simulink model "inc_enc_v26"  (R2023a)
settings: Solver=FixedStepDiscrete  StartTime=0.0  StopTime=SimulationsDauer  RelTol=1e-3
values from neighbouring files (symbols this model uses):
  CW_CCW_Switch = 0    [Init_IncreEncoder_v26.m]
  d_axis_hit_CompareValue = 125    [Init_IncreEncoder_v26.m]
  f_ISR = 40e3    (= 40000)    [Init_IncreEncoder_v26.m]
  IncPerTurn = 4100    [Init_IncreEncoder_v26.m]
  inital_zero_speed_timeout = speed_timeout_in_s*f_fpga    (= 5000)    [Init_IncreEncoder_v26.m]
  n_max = 6000    [Init_IncreEncoder_v26.m]
  Offset_Position_elec = 42    [Init_IncreEncoder_v26.m]
  Offset_Position_mech = 753    [Init_IncreEncoder_v26.m]
  OmegaPerOverSampl = 1500*((2*pi)/60)    (= 157.079632679)    [Init_IncreEncoder_v26.m]
  Periode = abs(1/Striche_pro_Sekunde)    [Init_IncreEncoder_v26.m]
  Phase_Delay_A = Periode/8    [Init_IncreEncoder_v26.m]
  Phase_Delay_B = -Periode/8    [Init_IncreEncoder_v26.m]
  PolePair = 10    [Init_IncreEncoder_v26.m]
  QuadratureFactor = 4    [Init_IncreEncoder_v26.m]
  reciprocal_iterations = 3    [Init_IncreEncoder_v26.m]
  T_fpga = 1/f_fpga    (= 1e-08)    [Init_IncreEncoder_v26.m]
  T_mech = 1e-08    [Init_IncreEncoder_v26.m]
undefined symbols (not defined in the file or in its folder): DiscIntNeverNeededParam
libraries: hdlsllib x4, dspsrcs4 x3, dspswit3 x2, spsEdgeDetectorLib x2, simulink_extras x1
(part 2 of 2)

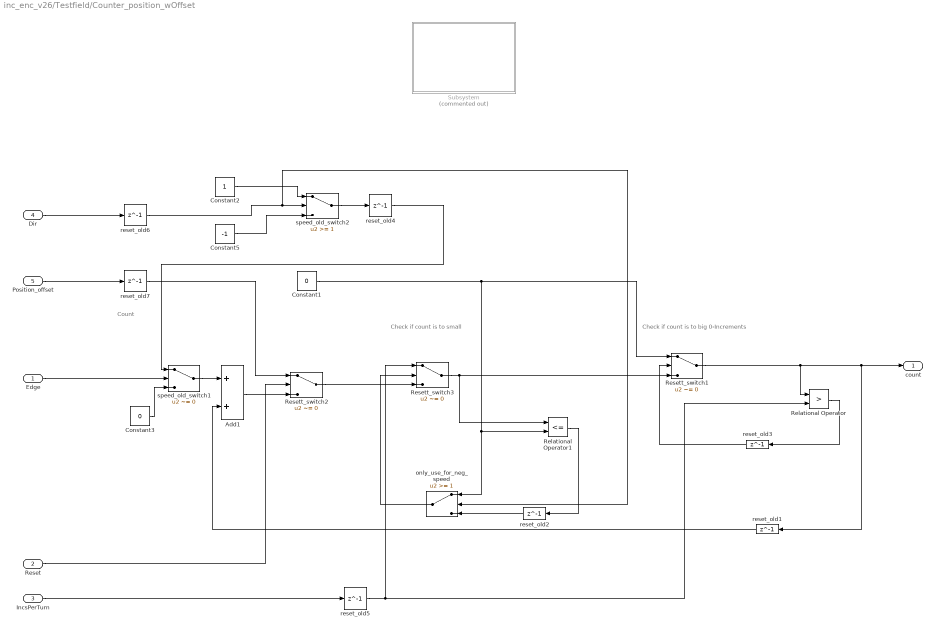
== system inc_enc_v26/Testfield/Counter_position_wOffset ==
  note: Check if count is to small
  note: Count
  note: Check if count is to big 0-Increments
  Edge : Inport
  Reset : Inport  Port=2
  IncsPerTurn : Inport  Port=3
  Dir : Inport  Port=4
  Position_offset : Inport  Port=5
  Add1 : Sum  AccumDataTypeStr=int16  OutDataTypeStr=int16
  Constant1 : Constant  Value=0  OutDataTypeStr=int16  SampleTime=-1
  Constant2 : Constant  OutDataTypeStr=int16  SampleTime=-1
  Constant3 : Constant  Value=0  OutDataTypeStr=int16  SampleTime=-1
  Constant5 : Constant  Value=-1  OutDataTypeStr=int16  SampleTime=-1
  Relational Operator : RelationalOperator  Operator=>  OutDataTypeStr=boolean  InputSameDT=off
  Relational Operator1 : RelationalOperator  Operator=<=  OutDataTypeStr=boolean  InputSameDT=off
  Resett_switch1 : Switch  Criteria=u2 ~= 0  OutDataTypeStr=uint16  SaturateOnIntegerOverflow=off  InputSameDT=off
  Resett_switch2 : Switch  Criteria=u2 ~= 0  OutDataTypeStr=int16  SaturateOnIntegerOverflow=off  InputSameDT=off
  Resett_switch3 : Switch  Criteria=u2 ~= 0  OutDataTypeStr=int16  SaturateOnIntegerOverflow=off  InputSameDT=off
  Subsystem : Subsystem  Commented=on
  only_use_for_neg_speed : Switch  Threshold=1  SaturateOnIntegerOverflow=off  InputSameDT=off
  reset_old{1..7} (7 alike) : Delay  DelayLength=1
  speed_old_switch1 : Switch  Criteria=u2 ~= 0  SaturateOnIntegerOverflow=off  InputSameDT=off
  speed_old_switch2 : Switch  Threshold=1  SaturateOnIntegerOverflow=off  InputSameDT=off
  count : Outport  VectorParamsAs1DForOutWhenUnconnected=off
  wires:
  speed_old_switch1/1 -> Add1/1
  Constant5/1 -> speed_old_switch2/3
  Relational Operator/1 -> reset_old3/1
  Constant2/1 -> speed_old_switch2/1
  reset_old4/1 -> speed_old_switch1/1
  reset_old5/1 -> Resett_switch3/1, Relational Operator/2
  Resett_switch2/1 -> Resett_switch3/3
  only_use_for_neg_speed/1 -> Resett_switch3/2
  Resett_switch3/1 -> Relational Operator1/1, Resett_switch1/3
  speed_old_switch2/1 -> reset_old4/1
  Relational Operator1/1 -> reset_old2/1
  reset_old3/1 -> Resett_switch1/2
  Resett_switch1/1 -> Relational Operator/1, count/1, reset_old1/1
  Constant1/1 -> only_use_for_neg_speed/1, Relational Operator1/2, Resett_switch1/1
  Constant3/1 -> speed_old_switch1/3
  IncsPerTurn/1 -> reset_old5/1
  Reset/1 -> Resett_switch2/2
  reset_old2/1 -> only_use_for_neg_speed/3
  Edge/1 -> speed_old_switch1/2
  reset_old1/1 -> Add1/2
  Position_offset/1 -> reset_old7/1
  Add1/1 -> Resett_switch2/3
  Dir/1 -> reset_old6/1
  reset_old6/1 -> only_use_for_neg_speed/2, speed_old_switch2/2
  reset_old7/1 -> Resett_switch2/1

== system inc_enc_v26/Testfield/Index_Latch ==
  Reset_in : Inport
  Constant : Constant  OutDataTypeStr=boolean
  Constant4 : Constant  Value=0  OutDataTypeStr=boolean
  Delay : Delay  DelayLength=1
  OR : Logic  Operator=OR  AllPortsSameDT=off  OutDataTypeStr=boolean
  Switch : Switch  Criteria=u2 > Threshold  SaturateOnIntegerOverflow=off  InputSameDT=off
  Index_found : Outport
  wires:
  Constant4/1 -> Switch/3
  Delay/1 -> OR/2
  Constant/1 -> Switch/1
  Switch/1 -> Index_found/1, Delay/1
  Reset_in/1 -> OR/1
  OR/1 -> Switch/2

== system inc_enc_v26/Create_Referenz/IncrementalEncoder_Floating/CutTheta_0_2PI ==
  In1 : Inport
  Add7 : Sum  Inputs=+-  OutDataTypeStr=double
  Gain : Gain  Gain=1/(2*pi)
  Gain11 : Gain  Gain=2*pi
  Rounding Function : Rounding
  Out1 : Outport  VectorParamsAs1DForOutWhenUnconnected=off
  wires:
  Gain/1 -> Rounding Function/1
  Rounding Function/1 -> Gain11/1
  Gain11/1 -> Add7/2
  In1/1 -> Gain/1, Add7/1
  Add7/1 -> Out1/1

== system inc_enc_v26/Create_Referenz/IncrementalEncoder_Floating/n_aus_theta_v4 ==
  theta : Inport
  Abs : Abs  SaturateOnIntegerOverflow=off
  Add : Sum  Inputs=-+
  Add1 : Sum  Inputs=+-
  Gain : Gain  Gain=2*pi
  Gain1 : Gain  Gain=1/T_mech
  Gain2 : Gain  Gain=60/(2*pi)
  Geschwindigkeitsfilter1 : Subsystem
  Rate Limiter2 1/T : RateLimiter  RisingSlewLimit=1/T_mech*10  FallingSlewLimit=-1/T_mech*10  SampleTimeMode=inherited
  Saturation : Saturate  UpperLimit=n_max  LowerLimit=-n_max
  Scope1 : Scope  NumInputPorts=5
  Scope2 : Scope  NumInputPorts=5
  Sign : Signum
  Switch : Switch  Threshold=3  SaturateOnIntegerOverflow=off  InputSameDT=off
  Unit Delay : UnitDelay  SampleTime=-1  HasFrameUpgradeWarning=on
  n : Outport  VectorParamsAs1DForOutWhenUnconnected=off
  wires:
  Switch/1 -> Scope1/3, Gain1/1
  Add/1 -> Scope2/1, Switch/1
  Gain/1 -> Add/1
  Sign/1 -> Gain/1
  Add1/1 -> Scope2/3, Add/2, Abs/1, Scope2/2, Switch/3, Sign/1
  Abs/1 -> Scope1/4, Switch/2
  Gain1/1 -> Scope1/2, Gain2/1
  theta/1 -> Scope2/5, Add1/1, Unit Delay/1
  Unit Delay/1 -> Scope2/4, Add1/2
  Gain2/1 -> Saturation/1
  Geschwindigkeitsfilter1/1(Out1) -> Scope1/5, Rate Limiter2 1/T/1
  Rate Limiter2 1/T/1 -> n/1
  Saturation/1 -> Scope1/1, Geschwindigkeitsfilter1/1(In1)

== system inc_enc_v26/IncEnc_V26/Counter_Theta_el_wOffset/Subsystem ==
  Add1 : Sum  AccumDataTypeStr=int16  OutDataTypeStr=int16
  Constant3 : Constant  Value=0  OutDataTypeStr=int16  SampleTime=-1
  Generate_Increment : Subsystem
  Resett_switch2 : Switch  Criteria=u2 ~= 0  OutDataTypeStr=int16  SaturateOnIntegerOverflow=off  InputSameDT=off
  reset_old6 : Delay  DelayLength=1
  speed_old_switch1 : Switch  Criteria=u2 ~= 0  SaturateOnIntegerOverflow=off  InputSameDT=off
  wires:
  ? -> speed_old_switch1/2
  ? -> Resett_switch2/2
  ? -> reset_old6/1
  ? -> Add1/2
  Generate_Increment/1(Increment) -> speed_old_switch1/1
  Resett_switch2/1 -> ?
  Constant3/1 -> speed_old_switch1/3
  ? -> Generate_Increment/1(Dir_in)
  reset_old6/1 -> Resett_switch2/1
  Add1/1 -> Resett_switch2/3
  speed_old_switch1/1 -> Add1/1

== system inc_enc_v26/IncEnc_V26/Counter_position_wOffset/Subsystem ==
  Add1 : Sum  AccumDataTypeStr=int16  OutDataTypeStr=int16
  Constant3 : Constant  Value=0  OutDataTypeStr=int16  SampleTime=-1
  Generate_Increment : Subsystem
  Resett_switch2 : Switch  Criteria=u2 ~= 0  OutDataTypeStr=int16  SaturateOnIntegerOverflow=off  InputSameDT=off
  reset_old6 : Delay  DelayLength=1
  speed_old_switch1 : Switch  Criteria=u2 ~= 0  SaturateOnIntegerOverflow=off  InputSameDT=off
  wires:
  speed_old_switch1/1 -> Add1/1
  Add1/1 -> Resett_switch2/3
  reset_old6/1 -> Resett_switch2/1
  ? -> Generate_Increment/1(Dir_in)
  Constant3/1 -> speed_old_switch1/3
  Resett_switch2/1 -> ?
  Generate_Increment/1(Increment) -> speed_old_switch1/1
  ? -> Add1/2
  ? -> reset_old6/1
  ? -> Resett_switch2/2
  ? -> speed_old_switch1/2

== system inc_enc_v26/IncEnc_V26/speed1/Average ==
  note: average 4 parallel measurements
  note: moving average of 4 last measurements, which in total results in a moving average of the last 8 samples
  "OmegaIn " : Inport
  NewMeasurement : Inport  Port=2
  DelayToCompensate_sum : Delay  DelayLength=1
  Demux2 : Demux
  Gain : Gain  Gain=1/4  OutDataTypeStr=fixdt(1,24,11)
  Gain1 : Gain  Gain=1/4  OutDataTypeStr=fixdt(1,24,11)
  Sum of Elements{1..6} (6 alike) : Sum  Inputs=2
  Unit Delay Enabled Synchronous : hdlsllib/Discrete/Unit Delay Enabled Synchronous  InitialCondition=0  SampleTime=-1
  Unit Delay Enabled Synchronous1 : hdlsllib/Discrete/Unit Delay Enabled Synchronous  InitialCondition=0  SampleTime=-1
  Unit Delay Enabled Synchronous2 : hdlsllib/Discrete/Unit Delay Enabled Synchronous  InitialCondition=0  SampleTime=-1
  delay : Delay  DelayLength=1
  delay1 : Delay  DelayLength=1
  Omega : Outport  VectorParamsAs1DForOutWhenUnconnected=off
  OmegaOut_MA_N4 : Outport  Port=2  VectorParamsAs1DForOutWhenUnconnected=off
  wires:
  Gain/1 -> OmegaOut_MA_N4/1  "omega moving average"
  DelayToCompensate_sum/1 -> Unit Delay Enabled Synchronous/1, delay1/1, Omega/1  "x(k)"
  Unit Delay Enabled Synchronous/1 -> Sum of Elements1/2, Unit Delay Enabled Synchronous1/1  "omega_delay1"
  Sum of Elements1/1 -> Sum of Elements3/1
  Sum of Elements3/1 -> Gain/1
  Unit Delay Enabled Synchronous2/1 -> Sum of Elements2/2  "omega_delay3"
  delay1/1 -> Sum of Elements1/1  "x(k)_1delayed"
  NewMeasurement/1 -> delay/1
  Sum of Elements2/1 -> Sum of Elements3/2
  delay/1 -> Unit Delay Enabled Synchronous/2, Unit Delay Enabled Synchronous1/2, Unit Delay Enabled Synchronous2/2  "enable_delayed"
  Unit Delay Enabled Synchronous1/1 -> Unit Delay Enabled Synchronous2/1, Sum of Elements2/1  "omega_delay2"
  Demux2/4 -> Sum of Elements5/2
  Demux2/3 -> Sum of Elements5/1
  Demux2/1 -> Sum of Elements4/1
  Sum of Elements5/1 -> Sum of Elements6/2
  Sum of Elements4/1 -> Sum of Elements6/1
  Demux2/2 -> Sum of Elements4/2
  Gain1/1 -> DelayToCompensate_sum/1  "omega summed 1/4"
  Sum of Elements6/1 -> Gain1/1
  "OmegaIn "/1 -> Demux2/1  "x(k)"

== system inc_enc_v26/IncEnc_V26/speed1/OS_factor_logic ==
  new_transisiton : Inport  PortDimensions=4
  Allow_ToCheckOversampling : Inport  Port=2
  state_edges : Inport  Port=3
  omega : Inport  Port=4
  OverSamplOmega : Inport  Port=5
  Abs : Abs  SaturateOnIntegerOverflow=off
  Constant : Constant  Commented=on  Value=[0,0,0,0]  OutDataTypeStr=boolean  SampleTime=T_fpga
  Data Type Conversion1 : DataTypeConversion  OutDataTypeStr=uint16  SaturateOnIntegerOverflow=off  RndMeth=Floor
  Delay1 : Delay  DelayLength=1  InitialCondition=0
  Delay6 : Delay  DelayLength=1  InitialCondition=0
  Delay7 : Delay  DelayLength=1  InitialCondition=1
  Sum : Sum  Inputs=+|-  AccumDataTypeStr=uint16
  align_oversamples : MATLAB Function  TreatAsAtomicUnit=on
  oversample_factor : MATLAB Function  TreatAsAtomicUnit=on
  oversampling_adjusted : Outport  PortDimensions=4
  oversampling_state : Outport  Port=2
  wires:
  OverSamplOmega/1 -> oversample_factor/3(OverSamplOmega)
  oversample_factor/1(state_Out) -> Delay7/1  "oversampling state Out"
  omega/1 -> Abs/1
  oversample_factor/2(InternalOmega_Out) -> Delay6/1
  Delay6/1 -> oversample_factor/5(InternalOmega)
  Abs/1 -> oversample_factor/2(ReadBack_Omega)
  Allow_ToCheckOversampling/1 -> oversample_factor/1(AllowCheckOverSampl)  "Allow_ToCheckOversampling"
  Delay7/1 -> Sum/1, align_oversamples/1(oversampling_factor), oversample_factor/4(state), Data Type Conversion1/1
  Data Type Conversion1/1 -> oversampling_state/1
  align_oversamples/1(delay_output) -> Delay1/1  "delay_output"
  new_transisiton/1 -> align_oversamples/2(new_transition)  "new_transistions"
  state_edges/1 -> align_oversamples/3(states)  "states"
  Sum/1 -> oversampling_adjusted/1
  Delay1/1 -> Sum/2

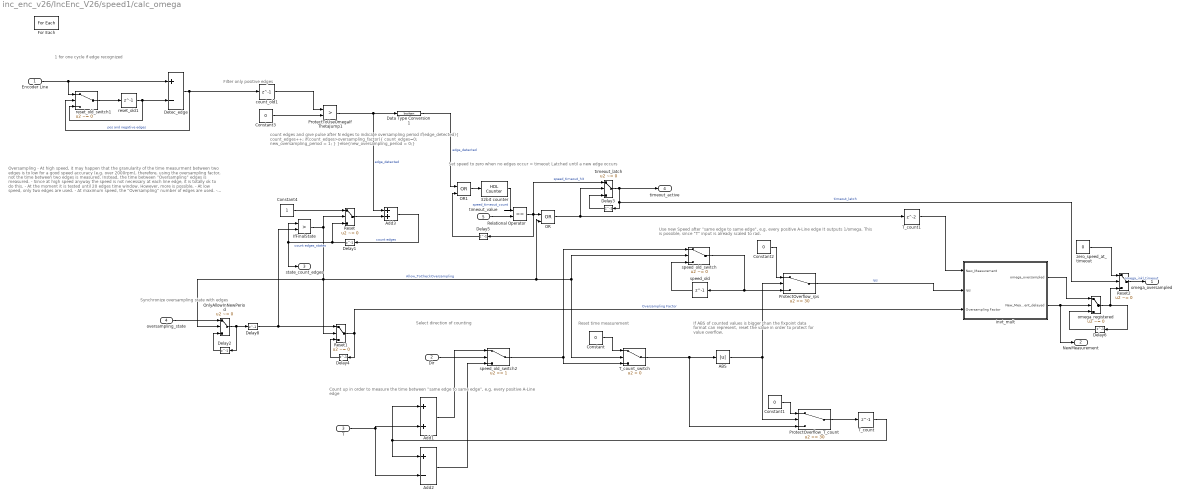
== system inc_enc_v26/IncEnc_V26/speed1/calc_omega ==
  note: Oversampling
      | - At high speed, it may happen that the granularity of the time measurment between
      | two edges is to low for a good speed accuracy (e.g. over 2000rpm), therefore, using
      | the oversampling factor, not the time between two edges is measured. Instead, the
      | time between "Oversampling" edges is measured.
      | - Since at high speed anyway the speed is not necessary at each line edge,
      |  it is totally ok to do this.
      | - At the moment it is tested until 20 edges time window. However, more is possible.
      | - At low speed, only two edges are used.
      | - At maximum speed, the "Oversampling" number of edges are used.
      | - Between them, a linear factor is used.
      | - Using the OverSampling number also at low speed is not possible,
      |  since the fixpoint range must be quite high! (fixdt(1,36,30) is used at the moment)
  note: Count up in order to measure the time between "same edge to same edge", e.g. every positive A-Line edge
  note: Reset time measurement
  note: 1 for one cycle if edge recognized
  note: Use new Speed after "same edge to same edge", e.g. every positive A-Line edge
      | It outputs 1/omega. This is possible, since "T" input is already scaled to rad.
  note: Select direction of counting
  note: If ABS of counted values is bigger than the
      | fixpoint data format can represent, reset the
      | value in order to protect for value overflow.
  note: Filter only positive edges
  note: count edges and give pulse after N edges to indicate oversampling period
      | if(edge_detected){
      | 	count_edges++;
      | 	if(count_edges>oversampling_factor){
      | 		count_edges=0;
      | 		new_oversampling_period = 1;
      | 	}
      | }else{new_oversampling_period = 0;}
  note: Synchronize oversampling state with edges
  note: Set speed to zero when no edges occur = timeout
      | Latched until a new edge occurs
  Encoder Line : Inport  Partition=on  PartitionDimension=1  PartitionWidth=1  PartitionOffset=0
  Dir : Inport  Port=2
  T : Inport  Port=3
  oversampling_state : Inport  Port=4  Partition=on  PartitionDimension=1  PartitionWidth=1  PartitionOffset=0
  timeout_value : Inport  Port=5  OutDataTypeStr=uint32
  32bit counter : hdlsllib/Sources/HDL Counter  CountType=Free running  CountInit=0  CountStep=1  CountMax=inital_zero_speed_timeout  CountFromType=Initial value  CountFrom=0  CountResetPort=on  CountLoadPort=off  CountEnbPort=off  CountDirPort=off  CountHitOutputPort=off  CountDataType=Unsigned  CountWordLen=32  CountFracLen=0  CountSampTime=1
  ABS : Abs  SaturateOnIntegerOverflow=off
  Add1 : Sum  OutDataTypeStr=Inherit: Same as first input
  Add2 : Sum  Inputs=+-  OutDataTypeStr=Inherit: Same as first input
  Add3 : Sum  OutDataTypeStr=Inherit: Same as accumulator
  Constant : Constant  Value=0  OutDataTypeStr=fixdt(1,38,32)  SampleTime=-1
  Constant1 : Constant  Value=0  OutDataTypeStr=fixdt(1,38,32)  SampleTime=-1
  Constant2 : Constant  Value=0  OutDataTypeStr=fixdt(1,38,32)  SampleTime=-1
  Constant3 : Constant  Value=0  OutDataTypeStr=int8  SampleTime=-1
  Constant4 : Constant  OutDataTypeStr=int8  SampleTime=-1
  Data Type Conversion1 : DataTypeConversion  OutDataTypeStr=boolean  SaturateOnIntegerOverflow=off  RndMeth=Floor
  Delay{1..6,8} (7 alike) : Delay  DelayLength=1  InitialCondition=0
  Detec_edge : Sum  Inputs=+-  AccumDataTypeStr=int8  OutDataTypeStr=int8
  For Each : ForEach  DisableCoverage=on
  IfFinalState : RelationalOperator  Operator=>  OutDataTypeStr=boolean  InputSameDT=off
  OR : Logic  Operator=OR  IconShape=distinctive  AllPortsSameDT=off  OutDataTypeStr=boolean
  OR1 : Logic  Operator=OR  IconShape=distinctive  AllPortsSameDT=off  OutDataTypeStr=boolean
  OnlyAllowInNewPeriod : Switch  Criteria=u2 ~= 0  Threshold=0.5  OutDataTypeStr=fixdt(0,16,0)  SaturateOnIntegerOverflow=off  InputSameDT=off
  ProtectOverflow_T_count : Switch  Threshold=30  SaturateOnIntegerOverflow=off  InputSameDT=off
  ProtectOverflow_rps : Switch  Threshold=30  OutDataTypeStr=fixdt(1,38,32)  SaturateOnIntegerOverflow=off  InputSameDT=off
  ProtectToUseOmegaIfThetaJump1 : RelationalOperator  Operator=>  OutDataTypeStr=fixdt(1,16)  InputSameDT=off
  Relational Operator : RelationalOperator  Operator===  OutDataTypeStr=boolean  RndMeth=Simplest  InputSameDT=off
  Reset : Switch  Criteria=u2 ~= 0  Threshold=0.5  OutDataTypeStr=fixdt(1,24,11)  SaturateOnIntegerOverflow=off  InputSameDT=off
  Reset1 : Switch  Criteria=u2 ~= 0  Threshold=0.5  OutDataTypeStr=Inherit: Inherit via back propagation  SaturateOnIntegerOverflow=off  InputSameDT=off
  Reset2 : Switch  Criteria=u2 ~= 0  Threshold=0.5  OutDataTypeStr=Inherit: Inherit via back propagation  SaturateOnIntegerOverflow=off  InputSameDT=off
  T_count : Delay  DelayLength=1
  T_count1 : Delay
  T_count_switch : Switch  Criteria=u2 > Threshold  SaturateOnIntegerOverflow=off  InputSameDT=off
  count_old1 : Delay  DelayLength=1
  invt_mult : Subsystem
  omega_registered : Switch  Criteria=u2 ~= 0  Threshold=0.5  SaturateOnIntegerOverflow=off  InputSameDT=off
  reset_old1 : Delay  DelayLength=1
  reset_old_switch1 : Switch  Criteria=u2 ~= 0  SaturateOnIntegerOverflow=off  InputSameDT=off
  speed_old : Delay  DelayLength=1
  speed_old_switch : Switch  Criteria=u2 ~= 0  OutDataTypeStr=fixdt(1,38,32)  SaturateOnIntegerOverflow=off  InputSameDT=off
  speed_old_switch2 : Switch  Threshold=1  SaturateOnIntegerOverflow=off  InputSameDT=off
  timeout_latch : Switch  Criteria=u2 ~= 0  Threshold=0.5  OutDataTypeStr=Inherit: Inherit via back propagation  SaturateOnIntegerOverflow=off  InputSameDT=off
  zero_speed_at_timeout : Constant  Value=0  OutDataTypeStr=fixdt(1,24,11)  SampleTime=-1
  omega_oversampled : Outport  ConcatenationDimension=1  VectorParamsAs1DForOutWhenUnconnected=off
  NewMeasurement : Outport  Port=2  ConcatenationDimension=1  VectorParamsAs1DForOutWhenUnconnected=off
  state_count_edges : Outport  Port=3  ConcatenationDimension=1  VectorParamsAs1DForOutWhenUnconnected=off
  timeout_active : Outport  Port=4  OutDataTypeStr=boolean  ConcatenationDimension=1  VectorParamsAs1DForOutWhenUnconnected=off
  wires:
  Constant/1 -> T_count_switch/1
  Constant1/1 -> ProtectOverflow_T_count/1
  Constant2/1 -> ProtectOverflow_rps/1
  speed_old_switch/1 -> ProtectOverflow_rps/3, speed_old/1
  speed_old/1 -> speed_old_switch/3
  T/1 -> Add1/2, Add2/2
  ProtectOverflow_T_count/1 -> T_count/1
  T_count/1 -> Add2/1, Add1/1
  speed_old_switch2/1 -> speed_old_switch/1, T_count_switch/3
  count_old1/1 -> ProtectToUseOmegaIfThetaJump1/1
  Constant3/1 -> ProtectToUseOmegaIfThetaJump1/2
  Encoder Line/1 -> reset_old_switch1/1, Detec_edge/1
  reset_old_switch1/1 -> reset_old1/1
  reset_old1/1 -> reset_old_switch1/3, Detec_edge/2
  Detec_edge/1 -> reset_old_switch1/2, count_old1/1  "pos and negative edges"
  Dir/1 -> speed_old_switch2/2
  Add1/1 -> speed_old_switch2/1
  Add2/1 -> speed_old_switch2/3
  T_count_switch/1 -> ABS/1, ProtectOverflow_T_count/3
  ABS/1 -> ProtectOverflow_T_count/2, ProtectOverflow_rps/2
  IfFinalState/1 -> OR/2, speed_old_switch/2, T_count_switch/2, Reset1/2, OnlyAllowInNewPeriod/2, Reset/2  "Allow_ToCheckOversampling"
  OnlyAllowInNewPeriod/1 -> Delay2/1, Delay8/1
  Delay1/1 -> Reset/3, state_count_edges/1, IfFinalState/1  "count edges_states"
  Add3/1 -> Delay1/1  "count edges"
  Reset/1 -> Add3/2
  Constant4/1 -> Reset/1
  Reset1/1 -> invt_mult/3(Oversampling Factor), Delay4/1  "Oversampling Factor"
  Delay2/1 -> OnlyAllowInNewPeriod/3
  oversampling_state/1 -> OnlyAllowInNewPeriod/1
  Delay4/1 -> Reset1/3
  Delay8/1 -> Reset1/1, IfFinalState/2
  ProtectToUseOmegaIfThetaJump1/1 -> Add3/1, Data Type Conversion1/1  "edge_detected"
  Relational Operator/1 -> Delay5/1, OR/1, timeout_latch/1  "speed_timeout_hit"
  zero_speed_at_timeout/1 -> Reset2/1
  Reset2/1 -> omega_oversampled/1  "omega_inkl_timeout"
  timeout_latch/1 -> timeout_active/1, Delay3/1, Reset2/2  "timeout_latch"
  Delay3/1 -> timeout_latch/3
  Data Type Conversion1/1 -> OR1/1  "edge_detected"
  timeout_value/1 -> Relational Operator/2
  32bit counter/1 -> Relational Operator/1  "speed_timeout_count"
  OR1/1 -> 32bit counter/1
  Delay5/1 -> OR1/2
  omega_registered/1 -> Reset2/3, Delay6/1
  Delay6/1 -> omega_registered/3
  OR/1 -> T_count1/1, timeout_latch/2
  ProtectOverflow_rps/1 -> invt_mult/2(rps)  "rps"
  invt_mult/1(omega_oversampled) -> omega_registered/1
  invt_mult/2(New_Measurement_delayed) -> NewMeasurement/1, omega_registered/2
  T_count1/1 -> invt_mult/1(New_Measurement)

== system inc_enc_v26/Testfield/Counter_position_wOffset/Subsystem ==
  Add1 : Sum  AccumDataTypeStr=int16  OutDataTypeStr=int16
  Constant3 : Constant  Value=0  OutDataTypeStr=int16  SampleTime=-1
  Generate_Increment : Subsystem
  Resett_switch2 : Switch  Criteria=u2 ~= 0  OutDataTypeStr=int16  SaturateOnIntegerOverflow=off  InputSameDT=off
  reset_old6 : Delay  DelayLength=1
  speed_old_switch1 : Switch  Criteria=u2 ~= 0  SaturateOnIntegerOverflow=off  InputSameDT=off
  wires:
  speed_old_switch1/1 -> Add1/1
  Add1/1 -> Resett_switch2/3
  reset_old6/1 -> Resett_switch2/1
  ? -> Generate_Increment/1(Dir_in)
  Constant3/1 -> speed_old_switch1/3
  Resett_switch2/1 -> ?
  Generate_Increment/1(Increment) -> speed_old_switch1/1
  ? -> Add1/2
  ? -> reset_old6/1
  ? -> Resett_switch2/2
  ? -> speed_old_switch1/2

== system inc_enc_v26/Create_Referenz/IncrementalEncoder_Floating/n_aus_theta_v4/Geschwindigkeitsfilter1 ==
  In1 : Inport
  Add1 : Sum  Inputs=+-
  Discrete-Time Integrator2 : DiscreteIntegrator  SampleTime=-1  ICPrevOutput=DiscIntNeverNeededParam  ICPrevScaledInput=DiscIntNeverNeededParam
  Gain2 2500 10000 : Gain  Gain=10000
  Scope1 : Scope  NumInputPorts=5
  Out1 : Outport  InitialOutput=[0]  VectorParamsAs1DForOutWhenUnconnected=off
  wires:
  Add1/1 -> Scope1/4, Gain2 2500 10000/1
  Gain2 2500 10000/1 -> Scope1/3, Discrete-Time Integrator2/1
  Discrete-Time Integrator2/1 -> Scope1/2, Out1/1, Add1/2
  In1/1 -> Scope1/5, Add1/1

== system inc_enc_v26/IncEnc_V26/Counter_Theta_el_wOffset/Subsystem/Generate_Increment ==
  Dir_in : Inport
  Constant2 : Constant  OutDataTypeStr=int16  SampleTime=-1
  Constant5 : Constant  Value=-1  OutDataTypeStr=int16  SampleTime=-1
  reset_old1 : Delay  DelayLength=1
  reset_old4 : Delay  DelayLength=1
  speed_old_switch2 : Switch  Threshold=1  SaturateOnIntegerOverflow=off  InputSameDT=off
  Increment : Outport
  wires:
  Dir_in/1 -> reset_old1/1
  reset_old4/1 -> Increment/1
  reset_old1/1 -> speed_old_switch2/2
  speed_old_switch2/1 -> reset_old4/1
  Constant2/1 -> speed_old_switch2/1
  Constant5/1 -> speed_old_switch2/3

== system inc_enc_v26/IncEnc_V26/Counter_position_wOffset/Subsystem/Generate_Increment ==
  Dir_in : Inport
  Constant2 : Constant  OutDataTypeStr=int16  SampleTime=-1
  Constant5 : Constant  Value=-1  OutDataTypeStr=int16  SampleTime=-1
  reset_old1 : Delay  DelayLength=1
  reset_old4 : Delay  DelayLength=1
  speed_old_switch2 : Switch  Threshold=1  SaturateOnIntegerOverflow=off  InputSameDT=off
  Increment : Outport
  wires:
  Constant5/1 -> speed_old_switch2/3
  Constant2/1 -> speed_old_switch2/1
  speed_old_switch2/1 -> reset_old4/1
  reset_old1/1 -> speed_old_switch2/2
  reset_old4/1 -> Increment/1
  Dir_in/1 -> reset_old1/1

== system inc_enc_v26/IncEnc_V26/speed1/calc_omega/invt_mult ==
  note: At high speed, e.g. at 6000rpm, an steady-state error occurs of around 2.5rpm. I would need more iterrations in the division to get it accurate.
      | However, i also tried to do a multiplication befor the division, so that the Oversampling factor do not gain the steady-state error.
      | But after a try, i still had a steady-state error, which was even bigger (3,2rpm). So i keep it so far.
      | However, the problem is not the fixed-point fromat. The problem is the number of itterations in the division!
      | This applies for 3 iterations
  note: Invert 1/omega and muliply with synchronized oversampling factor
  New_Measurement : Inport
  rps : Inport  Port=2
  Oversampling Factor : Inport  Port=3
  Data Type Conversion1 : DataTypeConversion  Commented=through  OutDataTypeStr=fixdt(1,24,11)  SaturateOnIntegerOverflow=off  RndMeth=Floor
  Data Type Conversion2 : DataTypeConversion  OutDataTypeStr=fixdt(1,24,12)  SaturateOnIntegerOverflow=off  RndMeth=Floor
  Data Type Conversion3 : DataTypeConversion  OutDataTypeStr=fixdt(0,6,0)  SaturateOnIntegerOverflow=off  RndMeth=Floor
  Data Type Conversion4 : DataTypeConversion  OutDataTypeStr=fixdt(1,32,18)  SaturateOnIntegerOverflow=off  RndMeth=Floor
  Div_i1 : Product  Inputs=**  OutDataTypeStr=fixdt(1,24,11)  RndMeth=Simplest  SaturateOnIntegerOverflow=on
  HDL Reciprocal : Reciprocal  NumberOfIterations=reciprocal_iterations
  omega_oversampled : Outport
  New_Measurement_delayed : Outport  Port=2
  wires:
  Oversampling Factor/1 -> Data Type Conversion3/1
  rps/1 -> Data Type Conversion4/1
  Data Type Conversion4/1 -> HDL Reciprocal/1  "before-invert"
  HDL Reciprocal/1 -> Data Type Conversion2/1  "after-invert"
  Data Type Conversion1/1 -> omega_oversampled/1
  Div_i1/1 -> Data Type Conversion1/1  "omega_oversampled"
  Data Type Conversion3/1 -> Div_i1/2  "before-invert"
  Data Type Conversion2/1 -> Div_i1/1  "omega/OS_factor"
  New_Measurement/1 -> New_Measurement_delayed/1

== system inc_enc_v26/Testfield/Counter_position_wOffset/Subsystem/Generate_Increment ==
  Dir_in : Inport
  Constant2 : Constant  OutDataTypeStr=int16  SampleTime=-1
  Constant5 : Constant  Value=-1  OutDataTypeStr=int16  SampleTime=-1
  reset_old1 : Delay  DelayLength=1
  reset_old4 : Delay  DelayLength=1
  speed_old_switch2 : Switch  Threshold=1  SaturateOnIntegerOverflow=off  InputSameDT=off
  Increment : Outport
  wires:
  Constant5/1 -> speed_old_switch2/3
  Constant2/1 -> speed_old_switch2/1
  speed_old_switch2/1 -> reset_old4/1
  reset_old1/1 -> speed_old_switch2/2
  reset_old4/1 -> Increment/1
  Dir_in/1 -> reset_old1/1

== matlab function inc_enc_v26/IncEnc_V26/speed1/OS_factor_logic/align_oversamples ==
  settings: fimath=fimath('RoundingMethod', 'Floor','OverflowAction', 'Wrap','ProductMode', 'FullPrecision', 'SumMode', 'FullPrecision')
  data: oversampling_factor input; new_transition input; states input; delay_output output
function delay_output  = fcn(oversampling_factor, new_transition, states)

% Fqint8 = fimath('RoundingMethod', 'Floor', 'OverflowAction', 'Wrap','ProductMode', 'SpecifyPrecision', 'ProductWordLength', 8,'ProductFractionLength',0,'SumMode','SpecifyPrecision','SumWordLength',8,'SumFractionLength',0);
half            = fi(0.5,false,1,1);
three_quarter   = fi(0.75,false,2,2);
persistent delay
if isempty(delay)
    delay    = logical([0 0 0 0]);
end

%% detect current ordering
if(new_transition(1) == 1) % omega_A updated
    
    %% change ordering
    %desired order when dir = +1: A, not B, not A, B => 1, 4, 3, 2
    %desired order when dir = -1: A, B, notA, not B  => 1, 2, 3, 4
    % desired order = omega1=A, omega2, omega3, omega4
    omega2= uint8(4);
    omega3= uint8(3);
    omega4= uint8(2);
    
    zero_logic = logical([0,0,0,0]);
    omega2_reset = zero_logic;
    omega3_reset = zero_logic;
    omega4_reset = zero_logic;
    
    omega2_reset(omega2) = true;
    omega3_reset(omega3) = true;
    omega4_reset(omega4) = true;
    
    omega2_target = uint8(oversampling_factor * half );
    omega3_target = uint8(oversampling_factor * three_quarter);
    omega4_target = uint8(oversampling_factor);
    
    if (oversampling_factor>=2)
        if (all(delay == 0) ) % no delay active
            
            if(states(omega4) ~= omega4_target)
                delay = omega4_reset;
                
            elseif(states(omega3) ~= omega3_target )
                delay = omega3_reset;
                
            elseif(states(omega2) ~= omega2_target )
                delay = omega2_reset;
                
            else
                delay = zero_logic; %final state is reached
            end
            
        else % a delay is already active
            if(         (delay(omega4) == 1 ) && (states(omega4) == (omega4_target-1) ) )
                delay = zero_logic;
            elseif(     (delay(omega3) == 1 ) && (states(omega3) == (omega3_target-1) ) )
                delay = zero_logic;
            %elseif(     isequal(delay, omega2_reset ) && (states(omega2) == (omega2_target-1) ) )
            elseif(     (delay(omega2) == 1 ) && (states(omega2) == (omega2_target-1) ) )
                delay = zero_logic;
            end
        end
    else
        delay = zero_logic;
    end
end

delay_output = delay;

end

== matlab function inc_enc_v26/IncEnc_V26/speed1/OS_factor_logic/oversample_factor ==
  settings: fimath=fimath('RoundingMethod', 'Floor','OverflowAction', 'Wrap','ProductMode', 'FullPrecision', 'SumMode', 'FullPrecision')
  data: AllowCheckOverSampl input; state_Out output fixdt(0,16,0); ReadBack_Omega input; OverSamplOmega input; state input fixdt(0,16,0); InternalOmega input; InternalOmega_Out output fixdt(1,24,11)
function [state_Out,InternalOmega_Out] = fcn(AllowCheckOverSampl, ReadBack_Omega,OverSamplOmega,state,InternalOmega)

Fq16    = fimath('RoundingMethod', 'Floor', 'OverflowAction', 'Wrap','ProductMode', 'FullPrecision', 'ProductWordLength', 16,'ProductFractionLength', 0,'SumMode','SpecifyPrecision','SumWordLength',16,'SumFractionLength',0);
Fq24    = fimath('RoundingMethod', 'Floor', 'OverflowAction', 'Wrap','ProductMode', 'FullPrecision', 'ProductWordLength', 24,'ProductFractionLength',11,'SumMode','SpecifyPrecision','SumWordLength',24,'SumFractionLength',11);

half    = fi(0.5,false,1,1);

if isempty(InternalOmega)
    InternalOmega = fi(0, 1, 24, 11);
end

%Counter State
if isempty(state)
    state = fi(1, 0, 16, 0);
end

%% Count Up 
% pre-calculate since used in comparison and assignment afterwards
Omega_ADD = fi(add(Fq24,InternalOmega,OverSamplOmega),1,24,11); 
Omega_SUB = fi(sub(Fq24,InternalOmega,OverSamplOmega),1,24,11);

if (ReadBack_Omega > Omega_ADD) && (AllowCheckOverSampl == 1)
    state= fi(add(Fq16,state,fi(1, 0, 16, 0)),0,16,0);   %Count up the measure-state
    InternalOmega = Omega_ADD;
elseif(ReadBack_Omega < Omega_SUB) && (AllowCheckOverSampl == 1)
    state= fi(sub(Fq16,state,fi(1, 0, 16, 0)),0,16,0);   %Count down the measure-state
    InternalOmega = Omega_SUB;
elseif(ReadBack_Omega < (OverSamplOmega*half)) && (AllowCheckOverSampl == 1)
    state = fi(1, 0, 16, 0);
end

%% Output the variables
state_Out = state;
InternalOmega_Out = InternalOmega;

end
